simulink library "mpclib"  (Simulink 6.0)
settings: Solver=ode45  SolverMode=SingleTasking  StartTime=0.0  StopTime=10.0  RelTol=1e-3
settings Model: Creator=jowen  LastModifiedBy=jowen
settings DataIOCC: SignalLoggingName=logsOut
settings OptimizationCC: BooleanDataType=off
settings DebuggingCC: CheckExecutionContextPreStartOutputMsg=on  CheckExecutionContextRuntimeOutputMsg=on  SolverPrmCheckMsg=none
settings HardwareCC: TargetUnknown=on
settings SFSimCC: SFSimApplyToAllLibs=on  SFSimBuildMode=Incremental

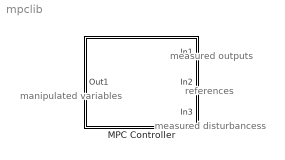
== system mpclib ==
  note: manipulated
      | variables
  note: measured
      | outputs
  note: references
  note: measured
      | disturbancess
  MPC Controller : Subsystem  Orientation=left  LoadFcn=mpc_block_resize  InitFcn=mpc_init  StartFcn=mpc_chkdimensions_sim  PropExecContextAcrossSSBoundary=on  mask(MPC){mpcobj=, n_mv=0, x0=[], ref_from_ws=off, ref_signal_name=[], ref_preview=on, md_from_ws=off, md_signal_name=[], md_preview=on, from_project=off, md_inport=on, project_file=MPCtask.mat, project_name=, task_name=}
      mask prompts: mpcobj "MPC Object"; n_mv "Starting Number of MVs"; x0 "Initial Extended State"; ref_from_ws "Reference from Workspace"; ref_signal_name "Reference"; ref_preview "Reference Preview"; md_from_ws "Measured Disturbance from workspace"; md_signal_name "Measured Disturbance"; md_preview "Measured Disturbance Preview"; from_project "Controller From Project"; md_inport "MD Signal"; project_file "Project File"; project_name "Project Name"; task_name "Task Name"
      mask init:
      | [ts,A,Cm,Dvm,Bu,Bv,PTYPE,nu,nv,nym,ny,nx,degrees,L,MuKduINV,KduINV,Kx,Ku1,Kut,Kr,Kv,zmin,rhsc0,Mlim,Mx,Mu1,Mv,rhsa0,TAB,optimalseq,utarget,lastx,lastu,p,Jm,DUFree,uoff,yoff,voff,myoff,no_md,no_ref,ref_from_ws,ref_signal,ref_preview,md_from_ws,md_signal,md_preview,maxiter,nxQP,openloopflag,md_inport,no_ym] = mpc_get_param_sim;
      | mpc_block_resize(gcb);
      settings: DeleteFcn=mpc_deletetask  OpenFcn=mpc_mask
      mask Display:
      | fprintf('MPC');
      | port_label('output', 1, 'mv')
      | port_label('input', 1, 'mo')
      | port_label('input', 2, 'ref')
      | port_label('input', 3, 'md')
      | port_label('input', 3, 'md')
      | port_label('input', 3, 'md')
      | port_label('input', 3, 'md')
      | port_label('input', 3, 'md')
      | port_label('input', 3, 'md')
      | port_label('input', 3, 'md')
      | port_label('input', 3, 'md')
      | port_label('input', 3, 'md')

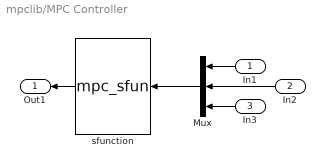
== system mpclib/MPC Controller ==
  In1 : Inport  Orientation=left  LatchInput=off
  In2 : Inport  Orientation=left  Port=2  LatchInput=off
  In3 : Inport  Orientation=left  Port=3  LatchInput=off
  Mux : Mux  Orientation=left  Inputs=3
  sfunction : S-Function  Orientation=left  FunctionName=mpc_sfun  Parameters=ts,A,Cm,Dvm,Bu,Bv,PTYPE,nu,nv,nym,ny,nx,degrees,L,MuKduINV,KduINV,Kx,Ku1,Kut,Kr,Kv,zmin,rhsc0,Mlim,Mx,Mu1,Mv,rhsa0,TAB,optimalseq,utarget,lastx,lastu,p,Jm,DUFree,uoff,yoff,voff,myoff,no_md,no_ref,ref_from_ws,ref_signal,ref_preview,md_from_ws,md_signal,md_preview,maxiter,nxQP,openloopflag,md_inport,no_ym
  Out1 : Outport  Orientation=left
  wires:
  Mux/1 -> sfunction/1
  In1/1 -> Mux/1
  sfunction/1 -> Out1/1
  In2/1 -> Mux/2
  In3/1 -> Mux/3
